simulink model "Nonlinear_Sim"  (R2019b)
settings: Solver=VariableStepAuto  StartTime=0.0  StopTime=30  RelTol=1e-3
settings Model: Creator=Ali Alaei  LastModifiedBy=Ali Alaei

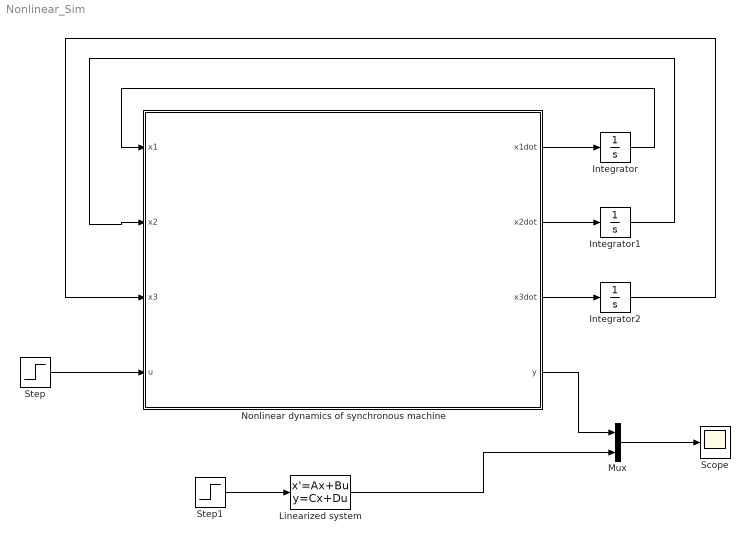
== system Nonlinear_Sim ==
  Integrator : Integrator  InitialCondition=0.5468
  Integrator1 : Integrator
  Integrator2 : Integrator  InitialCondition=9.6926
  Linearized system : StateSpace  A=[0 1 0;-77.3707 -0.2703 -6.2447;-0.9879 0 -0.322]  B=[0 0 1].'  C=[1 0 0]  D=0  InitialCondition=[0.5468 0 9.6926].'
  Mux : Mux  Inputs=2
  Nonlinear dynamics of synchronous machine : MATLAB Function  TreatAsAtomicUnit=on
  Scope : Scope
  Step : Step  Time=0  SampleTime=0
  Step1 : Step  Time=0  SampleTime=0
  wires:
  Nonlinear dynamics of synchronous machine/1(x1dot) -> Integrator/1
  Nonlinear dynamics of synchronous machine/2(x2dot) -> Integrator1/1
  Nonlinear dynamics of synchronous machine/3(x3dot) -> Integrator2/1
  Integrator/1 -> Nonlinear dynamics of synchronous machine/1(x1)
  Integrator1/1 -> Nonlinear dynamics of synchronous machine/2(x2)
  Integrator2/1 -> Nonlinear dynamics of synchronous machine/3(x3)
  Step/1 -> Nonlinear dynamics of synchronous machine/4(u)
  Step1/1 -> Linearized system/1
  Linearized system/1 -> Mux/2
  Mux/1 -> Scope/1
  Nonlinear dynamics of synchronous machine/4(y) -> Mux/1

== matlab function Nonlinear_Sim/Nonlinear dynamics of synchronous machine ==
  data: x1 input; x2 input; x3 input; x1dot output; x2dot output; x3dot output; u input; y output
function [x1dot,x2dot,x3dot,y] = fcn(x1,x2,x3,u)
x1dot=x2;
x2dot=-0.2703*x2+24.02*sin(2*x1)-12.01*x3*sin(x1);
x3dot=u-0.3222*x3+1.9*cos(x1);
y=x1;
end
